simulink model "Prp_TrqLeadCoord"  (R2016b)
settings: configuration reference "CodeGenConfigSet" (kept outside this file)
settings Model: Creator=wolf  LastModifiedBy=Wei Liang
settings ConfigSetRef: SourceLocation=Base Workspace

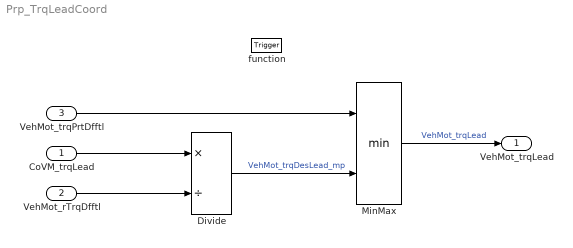
== system Prp_TrqLeadCoord ==
  CoVM_trqLead : Inport  Tag=Nm  Description=Propulsion torque after coordination with ESP interventions(wheel torque)  OutMin=-3000  OutMax=3000  OutDataTypeStr=Trq_Nm
  VehMot_rTrqDfftl : Inport  Description=Torque ratio of differential  Port=2  OutMin=-300  OutMax=300  OutDataTypeStr=TransRatio
  VehMot_trqPrtDfftl : Inport  Tag=Nm  Description=Differential protection torque  Port=3  OutMin=-3000  OutMax=3000  OutDataTypeStr=Trq_Nm
  function : TriggerPort  TriggerType=function-call  VariantControl=Variant
  Divide : Product  Inputs=*/  OutDataTypeStr=Trq_Nm
  MinMax : MinMax  Inputs=2  InputSameDT=on
  VehMot_trqLead : Outport  Tag=Nm  Description=Lead torque for propulsion (transmission output torque)  OutMin=-3000  OutMax=3000  OutDataTypeStr=Trq_Nm
  wires:
  VehMot_trqPrtDfftl/1 -> MinMax/1
  CoVM_trqLead/1 -> Divide/1
  Divide/1 -> MinMax/2  "VehMot_trqDesLead_mp"
  VehMot_rTrqDfftl/1 -> Divide/2
  MinMax/1 -> VehMot_trqLead/1  "VehMot_trqLead"
